simulink model "lab4"  (R2018a)
settings: Solver=VariableStepAuto  StartTime=0.0  StopTime=10  MaxStep=0.001  RelTol=1e-3
libraries: powerlib x5, ECEN315_Library x2, ECEN315_Library_Fault x1
settings Model: Creator=joshua  LastModifiedBy=joshua

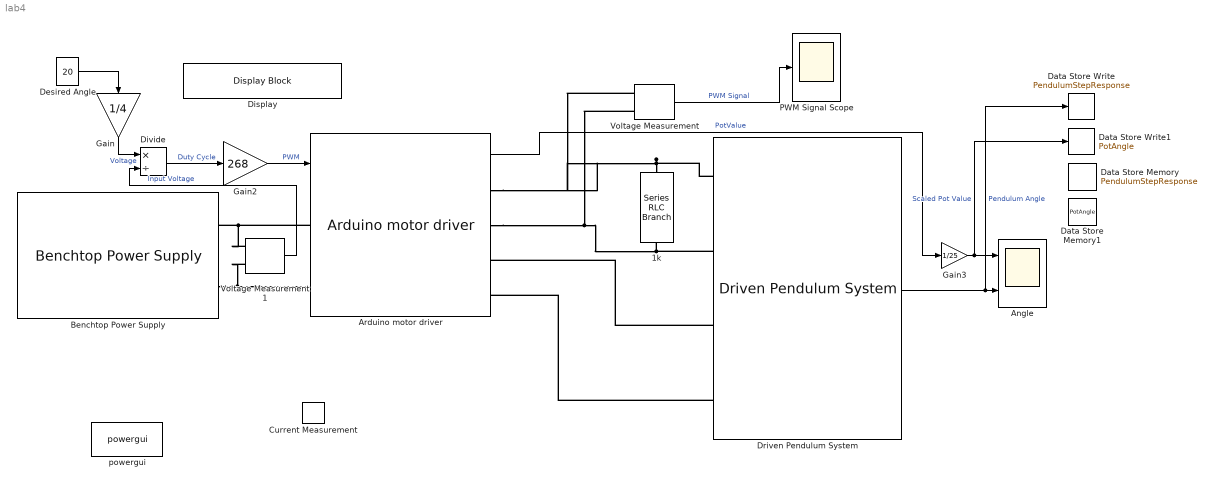
== system lab4 ==
  1k : powerlib/Elements/Series RLC Branch  LConnTagsString=__new0  RConnTagsString=__new0  BranchType=R  Resistance=1000  Inductance=1e-3  SetiL0=off  InitialCurrent=0  Capacitance=1e-6  Setx0=off  InitialVoltage=0  Measurements=None
  Angle : Scope  NumInputPorts=2
  Arduino motor driver : ECEN315_Library_Fault/Arduino motor driver  E=off
  Benchtop Power Supply : ECEN315_Library/Benchtop Power Supply  V=12
  Current Measurement : powerlib/Measurements/Current Measurement  PhasorSimulation=off  OutputType=Complex  PSBequivalent=0
  Data Store Memory : DataStoreMemory  DataStoreName=PendulumStepResponse  ReadBeforeWriteMsg=warning  WriteAfterWriteMsg=warning  WriteAfterReadMsg=warning  ShowAdditionalParam=off
  Data Store Memory1 : DataStoreMemory  DataStoreName=PotAngle  ReadBeforeWriteMsg=warning  WriteAfterWriteMsg=warning  WriteAfterReadMsg=warning  ShowAdditionalParam=off
  Data Store Write : DataStoreWrite  DataStoreName=PendulumStepResponse
  Data Store Write1 : DataStoreWrite  DataStoreName=PotAngle
  Desired Angle : Constant  Value=20  VectorParams1D=off  OutDataTypeStr=double
  Display : DisplayBlock  WebBlockId=38  LabelPosition=Hide
  Divide : Product  Inputs=*/
  Driven Pendulum System : ECEN315_Library/Driven Pendulum System  SystemSampleTime=-1
  Gain : Gain  Gain=1/4
  Gain2 : Gain  Gain=268
  Gain3 : Gain  Gain=1/25
  PWM Signal Scope : Scope
  Voltage Measurement : powerlib/Measurements/Voltage Measurement  PhasorSimulation=off  OutputType=Complex  PSBequivalent=0
  Voltage Measurement1 : powerlib/Measurements/Voltage Measurement  PhasorSimulation=off  OutputType=Complex  PSBequivalent=0
  powergui : powerlib/powergui  Priority=1  SimulationMode=Continuous  SampleTime=50e-6  frequency=60  Iterations=50  frequencyindice=0  Pbase=100e6  ErrMax=1e-4  UnitsV=kV  UnitsW=MW  buscounter=0  FunctionMessages=off  echomessages=off  EnableUseOfTLC=off  CurrentSourceSwitches=off  DisableSnubberDevices=off  DisableRonSwitches=off  DisableVfSwitches=off  DisplayEquations=off  SolverType=Tustin/Backward Euler (TBE)  Interpol=off  ExternalGateDelay=off  methode=off  Ts=100  x0status=blocks  SPID=on  SwTol=0  HookPort=off  RestoreLinks=warning  ResistiveCurrentMeasurement=off  Frange=[0:2:500]  Ylog=off  Xlog=on  ShowGrid=off  save=off  variable=ZData  structure=0  ZoomFFT=off  StartTime=0.0  cycles=1  DisplayStyle=1  fundamental=60  FreqAxis=off  MaxFrequency=1000  frequencyindicesteady=1  RmsSteady=1  display=off
  wires:
  Driven Pendulum System/1 -> Data Store Write/1, Angle/2  "Pendulum Angle"
  Desired Angle/1 -> Gain/1
  Gain3/1 -> Data Store Write1/1, Angle/1  "Scaled Pot Value"
  Arduino motor driver/1 -> Gain3/1  "PotValue"
  Voltage Measurement/1 -> PWM Signal Scope/1  "PWM Signal"
  Gain2/1 -> Arduino motor driver/1  "PWM"
  Voltage Measurement1/1 -> Divide/2  "Input Voltage"
  Divide/1 -> Gain2/1  "Duty Cycle"
  Gain/1 -> Divide/1  "Voltage"
  connections:
  1k/LConn1 -- Arduino motor driver/RConn1 -- Voltage Measurement/LConn1 -- Driven Pendulum System/LConn1
  Voltage Measurement/LConn2 -- 1k/RConn1 -- Driven Pendulum System/LConn2 -- Arduino motor driver/RConn2
  Arduino motor driver/LConn1 -- Voltage Measurement1/LConn1 -- Benchtop Power Supply/RConn1
  Benchtop Power Supply/RConn2 -- Voltage Measurement1/LConn2 -- Arduino motor driver/LConn2
  Driven Pendulum System/LConn3 -- Arduino motor driver/RConn3
  Driven Pendulum System/LConn4 -- Arduino motor driver/RConn4
